simulink model "RBCM_Model"  (R2023b)
settings: Solver=FixedStepAuto  StartTime=0.0  StopTime=10.0  RelTol=1e-3
PreLoadFcn:
  | % NXP_MBDT_S32K3 callback: DO NOT REMOVE
  | mbd_s32k3.common.nxp.model_callbacks.preLoadFcn();
PostLoadFcn:
  | % NXP_MBDT_S32K3 callback: DO NOT REMOVE
  | mbd_s32k3.common.nxp.model_callbacks.postLoadFcn();
InitFcn:
  | % NXP_MBDT_S32K3 callback: DO NOT REMOVE
  | mbd_s32k3.common.nxp.model_callbacks.initFcn();
undefined symbols (not defined in the file or in its folder): AccuFanPwr_hHsd3ch2, BspdPwr_lHsd1ch2, BuzzerPwr_lHsd3ch3, DevicePwr_12v_lHsd1ch1, DevicePwr_hHsd1ch2, DrsPwr_8v_lHsd3ch1, hHsd_Diagnose_AdcBuffer, ILPwr_hHsd1ch1, lHsd_Diagnose_AdcBuffer, LoggerPwr_lHsd1ch3, PumpFan1_hHsd4ch1, PumpFan2_hHsd4ch2, PumpPwr_hHsd3ch1, RGBLED0state, TaillightPwr_lHsd3ch4, TempSensorPwr_lHsd1ch4
libraries: mbd_s32k3_io_library x127, simulink x48, canmsglib x8, mbd_s32k3_communication_library x7, mbd_s32k3_isr_library x6, mbd_s32k3_cdd_library x3, mbd_s32k3_utility_library x1
(part 7 of 9)

== system RBCM_Model/HSD诊断分析子系统/Subsystem2 ==
  u1 : Inport
  Constant : Constant  Value=0xff  OutDataTypeStr=uint8
  Constant2 : Constant  Value=0  OutDataTypeStr=uint8
  Constant3 : Constant  OutDataTypeStr=uint8
  Constant4 : Constant  Value=2  OutDataTypeStr=uint8
  Gain : Gain  Gain=100
  Multiport Switch : MultiPortSwitch  DataPortOrder=Specify indices  DataPortIndices={0,5,90}  DataPortForDefault=Additional data port  DiagnosticForDefault=Warning  SaturateOnIntegerOverflow=off  InputSameDT=off
  u : Outport
  wires:
  Constant4/1 -> Multiport Switch/4
  Constant3/1 -> Multiport Switch/3
  Constant2/1 -> Multiport Switch/2
  Constant/1 -> Multiport Switch/5
  Multiport Switch/1 -> u/1
  Gain/1 -> Multiport Switch/1
  u1/1 -> Gain/1

== system RBCM_Model/HSD诊断分析子系统/Subsystem3 ==
  u1 : Inport
  Constant : Constant  Value=0xff  OutDataTypeStr=uint8
  Constant2 : Constant  Value=0  OutDataTypeStr=uint8
  Constant3 : Constant  OutDataTypeStr=uint8
  Constant4 : Constant  Value=2  OutDataTypeStr=uint8
  Gain : Gain  Gain=100
  Multiport Switch : MultiPortSwitch  DataPortOrder=Specify indices  DataPortIndices={0,5,90}  DataPortForDefault=Additional data port  DiagnosticForDefault=Warning  SaturateOnIntegerOverflow=off  InputSameDT=off
  u : Outport
  wires:
  Constant4/1 -> Multiport Switch/4
  Constant3/1 -> Multiport Switch/3
  Constant2/1 -> Multiport Switch/2
  Constant/1 -> Multiport Switch/5
  Multiport Switch/1 -> u/1
  Gain/1 -> Multiport Switch/1
  u1/1 -> Gain/1

== system RBCM_Model/HSD诊断分析子系统/Subsystem4 ==
  u1 : Inport
  Constant : Constant  Value=0xff  OutDataTypeStr=uint8
  Constant2 : Constant  Value=0  OutDataTypeStr=uint8
  Constant3 : Constant  OutDataTypeStr=uint8
  Constant4 : Constant  Value=2  OutDataTypeStr=uint8
  Gain : Gain  Gain=100
  Multiport Switch : MultiPortSwitch  DataPortOrder=Specify indices  DataPortIndices={0,5,90}  DataPortForDefault=Additional data port  DiagnosticForDefault=Warning  SaturateOnIntegerOverflow=off  InputSameDT=off
  u : Outport
  wires:
  u1/1 -> Gain/1
  Gain/1 -> Multiport Switch/1
  Multiport Switch/1 -> u/1
  Constant/1 -> Multiport Switch/5
  Constant2/1 -> Multiport Switch/2
  Constant3/1 -> Multiport Switch/3
  Constant4/1 -> Multiport Switch/4

== system RBCM_Model/HSD诊断分析子系统/Subsystem5 ==
  u1 : Inport
  Constant : Constant  Value=0xff  OutDataTypeStr=uint8
  Constant2 : Constant  Value=0  OutDataTypeStr=uint8
  Constant3 : Constant  OutDataTypeStr=uint8
  Constant4 : Constant  Value=2  OutDataTypeStr=uint8
  Gain : Gain  Gain=100
  Multiport Switch : MultiPortSwitch  DataPortOrder=Specify indices  DataPortIndices={0,5,90}  DataPortForDefault=Additional data port  DiagnosticForDefault=Warning  SaturateOnIntegerOverflow=off  InputSameDT=off
  u : Outport
  wires:
  Constant4/1 -> Multiport Switch/4
  Constant3/1 -> Multiport Switch/3
  Constant2/1 -> Multiport Switch/2
  Constant/1 -> Multiport Switch/5
  Multiport Switch/1 -> u/1
  Gain/1 -> Multiport Switch/1
  u1/1 -> Gain/1

== system RBCM_Model/HSD诊断分析子系统/Subsystem6 ==
  u1 : Inport
  Constant : Constant  Value=0xff  OutDataTypeStr=uint8
  Constant2 : Constant  Value=0  OutDataTypeStr=uint8
  Constant3 : Constant  OutDataTypeStr=uint8
  Constant4 : Constant  Value=2  OutDataTypeStr=uint8
  Gain : Gain  Gain=100
  Multiport Switch : MultiPortSwitch  DataPortOrder=Specify indices  DataPortIndices={0,5,290}  DataPortForDefault=Additional data port  DiagnosticForDefault=Warning  SaturateOnIntegerOverflow=off  InputSameDT=off
  u : Outport
  wires:
  u1/1 -> Gain/1
  Gain/1 -> Multiport Switch/1
  Multiport Switch/1 -> u/1
  Constant/1 -> Multiport Switch/5
  Constant2/1 -> Multiport Switch/2
  Constant3/1 -> Multiport Switch/3
  Constant4/1 -> Multiport Switch/4

== system RBCM_Model/HSD诊断分析子系统/Subsystem7 ==
  u1 : Inport
  Constant : Constant  Value=0xff  OutDataTypeStr=uint8
  Constant2 : Constant  Value=0  OutDataTypeStr=uint8
  Constant3 : Constant  OutDataTypeStr=uint8
  Constant4 : Constant  Value=2  OutDataTypeStr=uint8
  Gain : Gain  Gain=100
  Multiport Switch : MultiPortSwitch  DataPortOrder=Specify indices  DataPortIndices={0,5,290}  DataPortForDefault=Additional data port  DiagnosticForDefault=Warning  SaturateOnIntegerOverflow=off  InputSameDT=off
  u : Outport
  wires:
  u1/1 -> Gain/1
  Gain/1 -> Multiport Switch/1
  Multiport Switch/1 -> u/1
  Constant/1 -> Multiport Switch/5
  Constant2/1 -> Multiport Switch/2
  Constant3/1 -> Multiport Switch/3
  Constant4/1 -> Multiport Switch/4

== system RBCM_Model/HSD诊断分析子系统/Subsystem8 ==
  u1 : Inport
  Constant : Constant  Value=0xff  OutDataTypeStr=uint8
  Constant2 : Constant  Value=0  OutDataTypeStr=uint8
  Constant3 : Constant  OutDataTypeStr=uint8
  Constant4 : Constant  Value=2  OutDataTypeStr=uint8
  Gain : Gain  Gain=100
  Multiport Switch : MultiPortSwitch  DataPortOrder=Specify indices  DataPortIndices={0,5,290}  DataPortForDefault=Additional data port  DiagnosticForDefault=Warning  SaturateOnIntegerOverflow=off  InputSameDT=off
  u : Outport
  wires:
  Constant4/1 -> Multiport Switch/4
  Constant3/1 -> Multiport Switch/3
  Constant2/1 -> Multiport Switch/2
  Constant/1 -> Multiport Switch/5
  Multiport Switch/1 -> u/1
  Gain/1 -> Multiport Switch/1
  u1/1 -> Gain/1

== system RBCM_Model/HSD诊断分析子系统/Subsystem9 ==
  u1 : Inport
  Constant : Constant  Value=0xff  OutDataTypeStr=uint8
  Constant2 : Constant  Value=0  OutDataTypeStr=uint8
  Constant3 : Constant  OutDataTypeStr=uint8
  Constant4 : Constant  Value=2  OutDataTypeStr=uint8
  Gain : Gain  Gain=100
  Multiport Switch : MultiPortSwitch  DataPortOrder=Specify indices  DataPortIndices={0,5,290}  DataPortForDefault=Additional data port  DiagnosticForDefault=Warning  SaturateOnIntegerOverflow=off  InputSameDT=off
  u : Outport
  wires:
  u1/1 -> Gain/1
  Gain/1 -> Multiport Switch/1
  Multiport Switch/1 -> u/1
  Constant/1 -> Multiport Switch/5
  Constant2/1 -> Multiport Switch/2
  Constant3/1 -> Multiport Switch/3
  Constant4/1 -> Multiport Switch/4

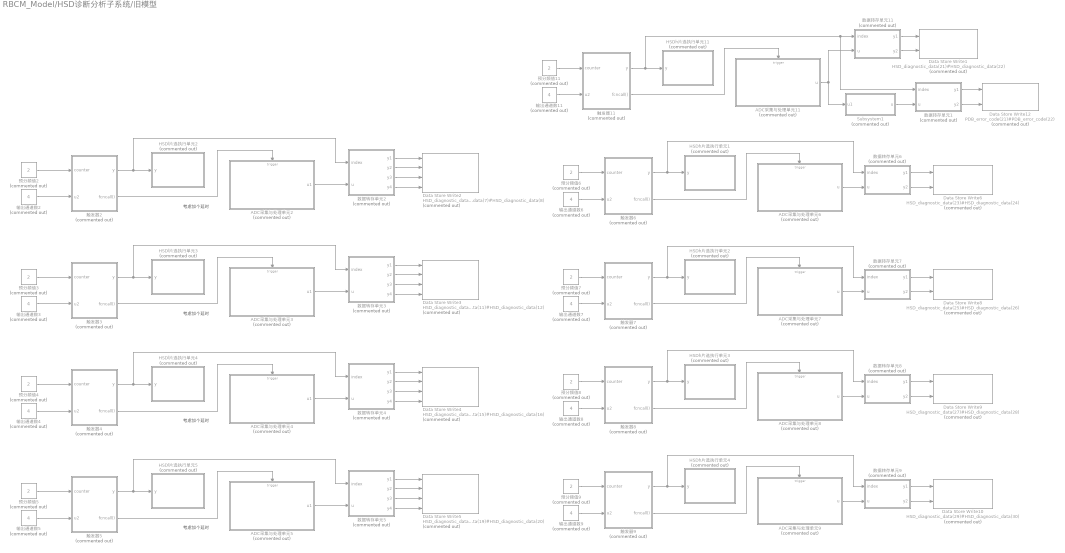
== system RBCM_Model/HSD诊断分析子系统/旧模型 ==
  note: 考虑加个延时
  note: 考虑加个延时
  note: 考虑加个延时
  note: 考虑加个延时
  ADC采集与处理单元11 : Subsystem  Commented=on
  ADC采集与处理单元2 : Subsystem  Commented=on
  ADC采集与处理单元3 : Subsystem  Commented=on
  ADC采集与处理单元4 : Subsystem  Commented=on
  ADC采集与处理单元5 : Subsystem  Commented=on
  ADC采集与处理单元6 : Subsystem  Commented=on
  ADC采集与处理单元7 : Subsystem  Commented=on
  ADC采集与处理单元8 : Subsystem  Commented=on
  ADC采集与处理单元9 : Subsystem  Commented=on
  Data Store Write1 : DataStoreWrite  Commented=on  DataStoreName=HSD_diagnostic_data  DataStoreElements=HSD_diagnostic_data(21)#HSD_diagnostic_data(22)  IndexOptions=Index vector (dialog)  Indices=1  OutputSizes=1
  Data Store Write10 : DataStoreWrite  Commented=on  DataStoreName=HSD_diagnostic_data  DataStoreElements=HSD_diagnostic_data(29)#HSD_diagnostic_data(30)  IndexOptions=Index vector (dialog)  Indices=1  OutputSizes=1
  Data Store Write12 : DataStoreWrite  Commented=on  DataStoreName=PDB_error_code  DataStoreElements=PDB_error_code(21)#PDB_error_code(22)  IndexOptions=Index vector (dialog)  Indices=1  OutputSizes=1
  Data Store Write2 : DataStoreWrite  Commented=on  DataStoreName=HSD_diagnostic_data  DataStoreElements=HSD_diagnostic_data(5)#HSD_diagnostic_data(6)#HSD_diagnostic_data(7)#HSD_diagnostic_data(8)  IndexOptions=Index vector (dialog)  Indices=1  OutputSizes=1
  Data Store Write3 : DataStoreWrite  Commented=on  DataStoreName=HSD_diagnostic_data  DataStoreElements=HSD_diagnostic_data(9)#HSD_diagnostic_data(10)#HSD_diagnostic_data(11)#HSD_diagnostic_data(12)  IndexOptions=Index vector (dialog)  Indices=1  OutputSizes=1
  Data Store Write4 : DataStoreWrite  Commented=on  DataStoreName=HSD_diagnostic_data  DataStoreElements=HSD_diagnostic_data(13)#HSD_diagnostic_data(14)#HSD_diagnostic_data(15)#HSD_diagnostic_data(16)  IndexOptions=Index vector (dialog)  Indices=1  OutputSizes=1
  Data Store Write5 : DataStoreWrite  Commented=on  DataStoreName=HSD_diagnostic_data  DataStoreElements=HSD_diagnostic_data(17)#HSD_diagnostic_data(18)#HSD_diagnostic_data(19)#HSD_diagnostic_data(20)  IndexOptions=Index vector (dialog)  Indices=1  OutputSizes=1
  Data Store Write6 : DataStoreWrite  Commented=on  DataStoreName=HSD_diagnostic_data  DataStoreElements=HSD_diagnostic_data(23)#HSD_diagnostic_data(24)  IndexOptions=Index vector (dialog)  Indices=1  OutputSizes=1
  Data Store Write8 : DataStoreWrite  Commented=on  DataStoreName=HSD_diagnostic_data  DataStoreElements=HSD_diagnostic_data(25)#HSD_diagnostic_data(26)  IndexOptions=Index vector (dialog)  Indices=1  OutputSizes=1
  Data Store Write9 : DataStoreWrite  Commented=on  DataStoreName=HSD_diagnostic_data  DataStoreElements=HSD_diagnostic_data(27)#HSD_diagnostic_data(28)  IndexOptions=Index vector (dialog)  Indices=1  OutputSizes=1
  HSDh片选执行单元1 : Subsystem  Commented=on
  HSDh片选执行单元11 : Subsystem  Commented=on
  HSDh片选执行单元2 : Subsystem  Commented=on
  HSDh片选执行单元3 : Subsystem  Commented=on
  HSDh片选执行单元4 : Subsystem  Commented=on
  HSDl片选执行单元2 : Subsystem  Commented=on
  HSDl片选执行单元3 : Subsystem  Commented=on
  HSDl片选执行单元4 : Subsystem  Commented=on
  HSDl片选执行单元5 : Subsystem  Commented=on
  Subsystem1 : Subsystem  Commented=on
  数据转存单元1 : MATLAB Function  Commented=on  TreatAsAtomicUnit=on
  数据转存单元11 : MATLAB Function  Commented=on  TreatAsAtomicUnit=on
  数据转存单元2 : MATLAB Function  Commented=on  TreatAsAtomicUnit=on
  数据转存单元3 : MATLAB Function  Commented=on  TreatAsAtomicUnit=on
  数据转存单元4 : MATLAB Function  Commented=on  TreatAsAtomicUnit=on
  数据转存单元5 : MATLAB Function  Commented=on  TreatAsAtomicUnit=on
  数据转存单元6 : MATLAB Function  Commented=on  TreatAsAtomicUnit=on
  数据转存单元7 : MATLAB Function  Commented=on  TreatAsAtomicUnit=on
  数据转存单元8 : MATLAB Function  Commented=on  TreatAsAtomicUnit=on
  数据转存单元9 : MATLAB Function  Commented=on  TreatAsAtomicUnit=on
  触发器11 : MATLAB Function  Commented=on  TreatAsAtomicUnit=on
  触发器2 : MATLAB Function  Commented=on  TreatAsAtomicUnit=on
  触发器3 : MATLAB Function  Commented=on  TreatAsAtomicUnit=on
  触发器4 : MATLAB Function  Commented=on  TreatAsAtomicUnit=on
  触发器5 : MATLAB Function  Commented=on  TreatAsAtomicUnit=on
  触发器6 : MATLAB Function  Commented=on  TreatAsAtomicUnit=on
  触发器7 : MATLAB Function  Commented=on  TreatAsAtomicUnit=on
  触发器8 : MATLAB Function  Commented=on  TreatAsAtomicUnit=on
  触发器9 : MATLAB Function  Commented=on  TreatAsAtomicUnit=on
  输出通道数{2..9,11} (9 alike) : Constant  Commented=on  Value=4  OutDataTypeStr=uint8
  预分频值{2..9,11} (9 alike) : Constant  Commented=on  Value=2  OutDataTypeStr=uint8
  wires:
  预分频值7/1 -> 触发器7/1(counter)
  ADC采集与处理单元3/1(u1) -> 数据转存单元3/2(u)
  输出通道数4/1 -> 触发器4/2(u2)
  触发器6/1(y) -> 数据转存单元6/1(index), HSDh片选执行单元1/1(y)
  预分频值8/1 -> 触发器8/1(counter)
  数据转存单元4/2(y2) -> Data Store Write4/2
  触发器8/1(y) -> 数据转存单元8/1(index), HSDh片选执行单元3/1(y)
  触发器7/2(fcncall()) -> ADC采集与处理单元7/Trigger
  数据转存单元3/4(y4) -> Data Store Write3/4
  数据转存单元3/1(y1) -> Data Store Write3/1
  数据转存单元4/3(y3) -> Data Store Write4/3
  触发器6/2(fcncall()) -> ADC采集与处理单元6/Trigger
  预分频值2/1 -> 触发器2/1(counter)
  预分频值6/1 -> 触发器6/1(counter)
  数据转存单元2/2(y2) -> Data Store Write2/2
  ADC采集与处理单元4/1(u1) -> 数据转存单元4/2(u)
  输出通道数8/1 -> 触发器8/2(u2)
  触发器2/2(fcncall()) -> ADC采集与处理单元2/Trigger
  输出通道数3/1 -> 触发器3/2(u2)
  数据转存单元2/1(y1) -> Data Store Write2/1
  触发器7/1(y) -> HSDh片选执行单元2/1(y), 数据转存单元7/1(index)
  触发器3/1(y) -> HSDl片选执行单元3/1(y), 数据转存单元3/1(index)
  输出通道数7/1 -> 触发器7/2(u2)
  触发器5/1(y) -> HSDl片选执行单元5/1(y), 数据转存单元5/1(index)
  触发器8/2(fcncall()) -> ADC采集与处理单元8/Trigger
  预分频值5/1 -> 触发器5/1(counter)
  ADC采集与处理单元5/1(u1) -> 数据转存单元5/2(u)
  数据转存单元6/1(y1) -> Data Store Write6/1
  预分频值4/1 -> 触发器4/1(counter)
  预分频值3/1 -> 触发器3/1(counter)
  数据转存单元3/2(y2) -> Data Store Write3/2
  数据转存单元7/2(y2) -> Data Store Write8/2
  输出通道数6/1 -> 触发器6/2(u2)
  触发器4/1(y) -> 数据转存单元4/1(index), HSDl片选执行单元4/1(y)
  输出通道数5/1 -> 触发器5/2(u2)
  数据转存单元9/2(y2) -> Data Store Write10/2
  ADC采集与处理单元8/1(u) -> 数据转存单元8/2(u)
  数据转存单元2/4(y4) -> Data Store Write2/4
  数据转存单元5/1(y1) -> Data Store Write5/1
  触发器2/1(y) -> 数据转存单元2/1(index), HSDl片选执行单元2/1(y)
  数据转存单元3/3(y3) -> Data Store Write3/3
  输出通道数2/1 -> 触发器2/2(u2)
  数据转存单元5/4(y4) -> Data Store Write5/4
  预分频值9/1 -> 触发器9/1(counter)
  数据转存单元2/3(y3) -> Data Store Write2/3
  ADC采集与处理单元2/1(u1) -> 数据转存单元2/2(u)
  ADC采集与处理单元9/1(u) -> 数据转存单元9/2(u)
  数据转存单元6/2(y2) -> Data Store Write6/2
  触发器4/2(fcncall()) -> ADC采集与处理单元4/Trigger
  ADC采集与处理单元6/1(u) -> 数据转存单元6/2(u)
  数据转存单元4/4(y4) -> Data Store Write4/4
  数据转存单元5/2(y2) -> Data Store Write5/2
  输出通道数9/1 -> 触发器9/2(u2)
  数据转存单元8/2(y2) -> Data Store Write9/2
  触发器9/1(y) -> HSDh片选执行单元4/1(y), 数据转存单元9/1(index)
  触发器5/2(fcncall()) -> ADC采集与处理单元5/Trigger
  触发器3/2(fcncall()) -> ADC采集与处理单元3/Trigger
  数据转存单元4/1(y1) -> Data Store Write4/1
  数据转存单元9/1(y1) -> Data Store Write10/1
  ADC采集与处理单元7/1(u) -> 数据转存单元7/2(u)
  数据转存单元7/1(y1) -> Data Store Write8/1
  数据转存单元8/1(y1) -> Data Store Write9/1
  触发器9/2(fcncall()) -> ADC采集与处理单元9/Trigger
  数据转存单元5/3(y3) -> Data Store Write5/3
  触发器11/2(fcncall()) -> ADC采集与处理单元11/Trigger
  数据转存单元1/2(y2) -> Data Store Write12/2
  Subsystem1/1(u) -> 数据转存单元1/2(u)
  数据转存单元11/2(y2) -> Data Store Write1/2
  数据转存单元11/1(y1) -> Data Store Write1/1
  输出通道数11/1 -> 触发器11/2(u2)
  预分频值11/1 -> 触发器11/1(counter)
  数据转存单元1/1(y1) -> Data Store Write12/1
  触发器11/1(y) -> HSDh片选执行单元11/1(y), 数据转存单元1/1(index), 数据转存单元11/1(index)
  ADC采集与处理单元11/1(u) -> Subsystem1/1(u1), 数据转存单元11/2(u)

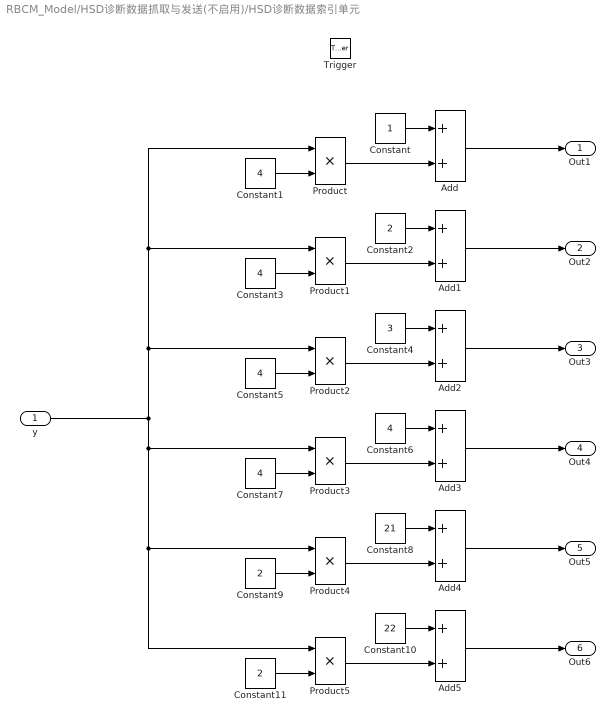
== system RBCM_Model/HSD诊断数据抓取与发送(不启用)/HSD诊断数据索引单元 ==
  y : Inport  OutDataTypeStr=uint8
  Trigger : TriggerPort  TriggerType=function-call  VariantControl=(inherit)  PortDimensions=1
  Add{,1..5} (6 alike) : Sum  OutDataTypeStr=uint8
  Constant : Constant  OutDataTypeStr=uint8
  Constant{1,3,5..7} (5 alike) : Constant  Value=4  OutDataTypeStr=uint8
  Constant10 : Constant  Value=22  OutDataTypeStr=uint8
  Constant11 : Constant  Value=2  OutDataTypeStr=uint8
  Constant2 : Constant  Value=2  OutDataTypeStr=uint8
  Constant4 : Constant  Value=3  OutDataTypeStr=uint8
  Constant8 : Constant  Value=21  OutDataTypeStr=uint8
  Constant9 : Constant  Value=2  OutDataTypeStr=uint8
  Product{,1..5} (6 alike) : Product  OutDataTypeStr=uint8
  Out1 : Outport  OutDataTypeStr=uint8
  Out2 : Outport  Port=2  OutDataTypeStr=uint8
  Out3 : Outport  Port=3  OutDataTypeStr=uint8
  Out4 : Outport  Port=4  OutDataTypeStr=uint8
  Out5 : Outport  Port=5  OutDataTypeStr=uint8
  Out6 : Outport  Port=6  OutDataTypeStr=uint8
  wires:
  Product/1 -> Add/2
  Constant1/1 -> Product/2
  Add/1 -> Out1/1
  Constant/1 -> Add/1
  Constant2/1 -> Add1/1
  Add1/1 -> Out2/1
  Constant3/1 -> Product1/2
  Product1/1 -> Add1/2
  Product3/1 -> Add3/2
  Constant7/1 -> Product3/2
  Add3/1 -> Out4/1
  Constant6/1 -> Add3/1
  Constant4/1 -> Add2/1
  Add2/1 -> Out3/1
  Constant5/1 -> Product2/2
  Product2/1 -> Add2/2
  Product4/1 -> Add4/2
  Constant9/1 -> Product4/2
  Add4/1 -> Out5/1
  Constant8/1 -> Add4/1
  Constant10/1 -> Add5/1
  Add5/1 -> Out6/1
  Constant11/1 -> Product5/2
  Product5/1 -> Add5/2
  y/1 -> Product5/1, Product4/1, Product3/1, Product2/1, Product1/1, Product/1

== system RBCM_Model/HSD驱动子系统/HSDh输出控制单元1 ==
  In1 : Inport
  In2 : Inport  Port=2
  Dio : mbd_s32k3_io_library/Dio  Commented=on  api_func=Dio_WriteChannel  channel=RGBLED0_BLUE  channel_group=No channel groups configured  port=PTB_H  gpioSim=on  text=<binary blob, 15246 chars, not shown>
      settings: SourceProductName=NXP Model-Based Design Toolbox for S32K3 MCUs
  Dio1 : mbd_s32k3_io_library/Dio  api_func=Dio_WriteChannel  channel=RGBLED0_BLUE  channel_group=No channel groups configured  port=PTB_H  gpioSim=on  text=<binary blob, 15399 chars, not shown>
      settings: SourceProductName=NXP Model-Based Design Toolbox for S32K3 MCUs
  wires:
  In2/1 -> Dio1/1
  In1/1 -> Dio/1

== system RBCM_Model/HSD驱动子系统/HSDh输出控制单元2 ==
  note: PUMP_PWM_CTRL
  In1 : Inport  OutDataTypeStr=uint8
  In2 : Inport  Port=2  OutDataTypeStr=uint8
  Dio : mbd_s32k3_io_library/Dio  api_func=Dio_WriteChannel  channel=RGBLED0_BLUE  channel_group=No channel groups configured  port=PTB_H  gpioSim=on  text=<binary blob, 15399 chars, not shown>
      settings: SourceProductName=NXP Model-Based Design Toolbox for S32K3 MCUs
  Dio1 : mbd_s32k3_io_library/Dio  api_func=Dio_WriteChannel  channel=RGBLED0_BLUE  channel_group=No channel groups configured  port=PTB_H  gpioSim=on  text=<binary blob, 15399 chars, not shown>
      settings: SourceProductName=NXP Model-Based Design Toolbox for S32K3 MCUs
  wires:
  In2/1 -> Dio1/1
  In1/1 -> Dio/1

== system RBCM_Model/HSD驱动子系统/HSDh输出控制单元3 ==
  note: FAN1_PWM_CTRL
  In1 : Inport
  In2 : Inport  Port=2
  Dio : mbd_s32k3_io_library/Dio  api_func=Dio_WriteChannel  channel=RGBLED0_BLUE  channel_group=No channel groups configured  port=PTB_H  gpioSim=on  text=<binary blob, 15399 chars, not shown>
      settings: SourceProductName=NXP Model-Based Design Toolbox for S32K3 MCUs
  Dio1 : mbd_s32k3_io_library/Dio  api_func=Dio_WriteChannel  channel=RGBLED0_BLUE  channel_group=No channel groups configured  port=PTB_H  gpioSim=on  text=<binary blob, 15399 chars, not shown>
      settings: SourceProductName=NXP Model-Based Design Toolbox for S32K3 MCUs
  wires:
  In2/1 -> Dio1/1
  In1/1 -> Dio/1

== system RBCM_Model/HSD驱动子系统/HSDh输出控制单元4 ==
  note: FAN1_PWM_CTRL
  In1 : Inport
  In2 : Inport  Port=2
  Dio : mbd_s32k3_io_library/Dio  api_func=Dio_WriteChannel  channel=RGBLED0_BLUE  channel_group=No channel groups configured  port=PTB_H  gpioSim=on  text=<binary blob, 15399 chars, not shown>
      settings: SourceProductName=NXP Model-Based Design Toolbox for S32K3 MCUs
  Dio1 : mbd_s32k3_io_library/Dio  api_func=Dio_WriteChannel  channel=RGBLED0_BLUE  channel_group=No channel groups configured  port=PTB_H  gpioSim=on  text=<binary blob, 15399 chars, not shown>
      settings: SourceProductName=NXP Model-Based Design Toolbox for S32K3 MCUs
  wires:
  In2/1 -> Dio1/1
  In1/1 -> Dio/1

== system RBCM_Model/HSD驱动子系统/HSDh输出控制单元5 ==
  In1 : Inport
  In2 : Inport  Port=2
  Dio : mbd_s32k3_io_library/Dio  api_func=Dio_WriteChannel  channel=RGBLED0_BLUE  channel_group=No channel groups configured  port=PTB_H  gpioSim=on  text=<binary blob, 15399 chars, not shown>
      settings: SourceProductName=NXP Model-Based Design Toolbox for S32K3 MCUs
  Dio1 : mbd_s32k3_io_library/Dio  api_func=Dio_WriteChannel  channel=RGBLED0_BLUE  channel_group=No channel groups configured  port=PTB_H  gpioSim=on  text=<binary blob, 15399 chars, not shown>
      settings: SourceProductName=NXP Model-Based Design Toolbox for S32K3 MCUs
  wires:
  In2/1 -> Dio1/1
  In1/1 -> Dio/1

== system RBCM_Model/HSD驱动子系统/HSDh输出控制单元6 ==
  In1 : Inport
  In2 : Inport  Port=2
  Dio : mbd_s32k3_io_library/Dio  api_func=Dio_WriteChannel  channel=RGBLED0_BLUE  channel_group=No channel groups configured  port=PTB_H  gpioSim=on  text=<binary blob, 15399 chars, not shown>
      settings: SourceProductName=NXP Model-Based Design Toolbox for S32K3 MCUs
  Dio1 : mbd_s32k3_io_library/Dio  api_func=Dio_WriteChannel  channel=RGBLED0_BLUE  channel_group=No channel groups configured  port=PTB_H  gpioSim=on  text=<binary blob, 15399 chars, not shown>
      settings: SourceProductName=NXP Model-Based Design Toolbox for S32K3 MCUs
  wires:
  In1/1 -> Dio/1
  In2/1 -> Dio1/1

== system RBCM_Model/HSD驱动子系统/HSDl输出控制单元1 ==
  In1 : Inport
  In2 : Inport  Port=2
  In3 : Inport  Port=3
  In6 : Inport  Port=4
  Dio{,1..3} (4 alike) : mbd_s32k3_io_library/Dio  api_func=Dio_WriteChannel  channel=RGBLED0_BLUE  channel_group=No channel groups configured  port=PTB_H  gpioSim=on  text=<binary blob, 15399 chars, not shown>
      settings: SourceProductName=NXP Model-Based Design Toolbox for S32K3 MCUs
  wires:
  In6/1 -> Dio3/1
  In2/1 -> Dio1/1
  In3/1 -> Dio2/1
  In1/1 -> Dio/1

== system RBCM_Model/HSD驱动子系统/HSDl输出控制单元2 ==
  In1 : Inport
  In2 : Inport  Port=2
  In3 : Inport  Port=3
  In6 : Inport  Port=4
  Dio{,1,3..4} (4 alike) : mbd_s32k3_io_library/Dio  api_func=Dio_WriteChannel  channel=RGBLED0_BLUE  channel_group=No channel groups configured  port=PTB_H  gpioSim=on  text=<binary blob, 15399 chars, not shown>
      settings: SourceProductName=NXP Model-Based Design Toolbox for S32K3 MCUs
  wires:
  In1/1 -> Dio/1
  In3/1 -> Dio4/1
  In2/1 -> Dio1/1
  In6/1 -> Dio3/1

== system RBCM_Model/HSD驱动子系统/HSDl输出控制单元3 ==
  In1 : Inport
  In2 : Inport  Port=2
  In3 : Inport  Port=3
  In6 : Inport  Port=4
  Dio{,1..3} (4 alike) : mbd_s32k3_io_library/Dio  api_func=Dio_WriteChannel  channel=RGBLED0_BLUE  channel_group=No channel groups configured  port=PTB_H  gpioSim=on  text=<binary blob, 15399 chars, not shown>
      settings: SourceProductName=NXP Model-Based Design Toolbox for S32K3 MCUs
  wires:
  In6/1 -> Dio3/1
  In2/1 -> Dio1/1
  In3/1 -> Dio2/1
  In1/1 -> Dio/1

== system RBCM_Model/HSD驱动子系统/HSDl输出控制单元4 ==
  In1 : Inport
  In2 : Inport  Port=2
  In3 : Inport  Port=3
  In6 : Inport  Port=4
  Dio{,1..3} (4 alike) : mbd_s32k3_io_library/Dio  api_func=Dio_WriteChannel  channel=RGBLED0_BLUE  channel_group=No channel groups configured  port=PTB_H  gpioSim=on  text=<binary blob, 15399 chars, not shown>
      settings: SourceProductName=NXP Model-Based Design Toolbox for S32K3 MCUs
  wires:
  In1/1 -> Dio/1
  In3/1 -> Dio2/1
  In2/1 -> Dio1/1
  In6/1 -> Dio3/1

== system RBCM_Model/HSD驱动子系统/HSDl输出控制单元5 ==
  In1 : Inport
  In2 : Inport  Port=2
  In3 : Inport  Port=3
  In6 : Inport  Port=4
  Dio{,1..3} (4 alike) : mbd_s32k3_io_library/Dio  api_func=Dio_WriteChannel  channel=RGBLED0_BLUE  channel_group=No channel groups configured  port=PTB_H  gpioSim=on  text=<binary blob, 15399 chars, not shown>
      settings: SourceProductName=NXP Model-Based Design Toolbox for S32K3 MCUs
  wires:
  In6/1 -> Dio3/1
  In2/1 -> Dio1/1
  In3/1 -> Dio2/1
  In1/1 -> Dio/1

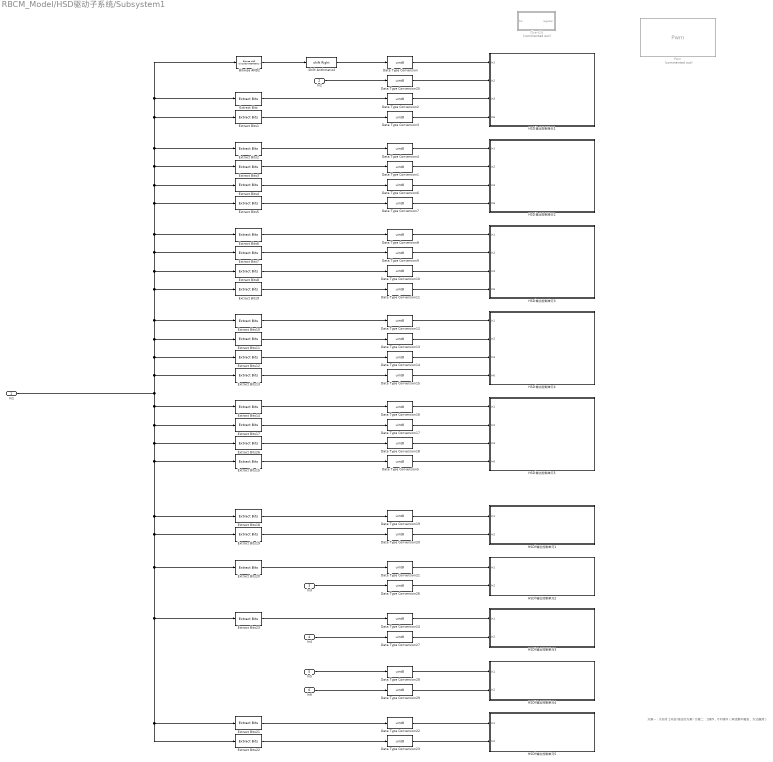
== system RBCM_Model/HSD驱动子系统/Subsystem1 ==
  note: 方案一：0关闭 1开启(现在的方案)
      | 方案二：1操作，0不操作（异或集中触发，方式最简）
  In1 : Inport  OutDataTypeStr=uint32
  In2 : Inport  Port=2  OutDataTypeStr=uint8
  In3 : Inport  Port=3  OutDataTypeStr=uint8
  In4 : Inport  Port=4  OutDataTypeStr=uint8
  In5 : Inport  Port=5  OutDataTypeStr=uint8
  In6 : Inport  Port=6  OutDataTypeStr=uint8
  Bitwise AND2 : simulink/Logic and Bit Operations/Bitwise Operator  logicop=AND  UseBitMask=on  BitMask=bin2dec('00000001')  BitMaskRealWorld=Stored Integer
      settings: LibrarySourceBlock=|
      | simulink/Quick Insert/Logic and Bit
      | Operations/Bitwise AND
  Chart19 : Stateflow chart  Commented=on  TreatAsAtomicUnit=on
  Data Type Conversion{,1..29} (30 alike) : DataTypeConversion  OutDataTypeStr=uint8  SaturateOnIntegerOverflow=off  RndMeth=Floor
  Extract Bits : simulink/Logic and Bit Operations/Extract Bits  bitsToExtract=Range of bits  numBits=8  bitIdxRange=[2 2]  outScalingMode=Preserve fixed-point scaling
  Extract Bits1 : simulink/Logic and Bit Operations/Extract Bits  bitsToExtract=Range of bits  numBits=8  bitIdxRange=[3 3]  outScalingMode=Preserve fixed-point scaling
  Extract Bits10 : simulink/Logic and Bit Operations/Extract Bits  bitsToExtract=Range of bits  numBits=8  bitIdxRange=[24 25]  outScalingMode=Preserve fixed-point scaling
  Extract Bits11 : simulink/Logic and Bit Operations/Extract Bits  bitsToExtract=Range of bits  numBits=8  bitIdxRange=[26 27]  outScalingMode=Preserve fixed-point scaling
  Extract Bits12 : simulink/Logic and Bit Operations/Extract Bits  bitsToExtract=Range of bits  numBits=8  bitIdxRange=[28 29]  outScalingMode=Preserve fixed-point scaling
  Extract Bits13 : simulink/Logic and Bit Operations/Extract Bits  bitsToExtract=Range of bits  numBits=8  bitIdxRange=[30 31]  outScalingMode=Preserve fixed-point scaling
  Extract Bits14 : simulink/Logic and Bit Operations/Extract Bits  bitsToExtract=Range of bits  numBits=8  bitIdxRange=[32 33]  outScalingMode=Preserve fixed-point scaling
  Extract Bits{15,18..23,26} (8 alike) : simulink/Logic and Bit Operations/Extract Bits  bitsToExtract=Range of bits  numBits=8  bitIdxRange=[36 37]  outScalingMode=Preserve fixed-point scaling
  Extract Bits17 : simulink/Logic and Bit Operations/Extract Bits  bitsToExtract=Range of bits  numBits=8  bitIdxRange=[34 35]  outScalingMode=Preserve fixed-point scaling
  Extract Bits2 : simulink/Logic and Bit Operations/Extract Bits  bitsToExtract=Range of bits  numBits=8  bitIdxRange=[4 4]  outScalingMode=Preserve fixed-point scaling
  Extract Bits3 : simulink/Logic and Bit Operations/Extract Bits  bitsToExtract=Range of bits  numBits=8  bitIdxRange=[5 5]  outScalingMode=Preserve fixed-point scaling
  Extract Bits4 : simulink/Logic and Bit Operations/Extract Bits  bitsToExtract=Range of bits  numBits=8  bitIdxRange=[6 6]  outScalingMode=Preserve fixed-point scaling
  Extract Bits5 : simulink/Logic and Bit Operations/Extract Bits  bitsToExtract=Range of bits  numBits=8  bitIdxRange=[7 7]  outScalingMode=Preserve fixed-point scaling
  Extract Bits6 : simulink/Logic and Bit Operations/Extract Bits  bitsToExtract=Range of bits  numBits=8  bitIdxRange=[16 17]  outScalingMode=Preserve fixed-point scaling
  Extract Bits7 : simulink/Logic and Bit Operations/Extract Bits  bitsToExtract=Range of bits  numBits=8  bitIdxRange=[18 19]  outScalingMode=Preserve fixed-point scaling
  Extract Bits8 : simulink/Logic and Bit Operations/Extract Bits  bitsToExtract=Range of bits  numBits=8  bitIdxRange=[20 21]  outScalingMode=Preserve fixed-point scaling
  Extract Bits9 : simulink/Logic and Bit Operations/Extract Bits  bitsToExtract=Range of bits  numBits=8  bitIdxRange=[22 23]  outScalingMode=Preserve fixed-point scaling
  HSDh输出控制单元1 : Subsystem
  HSDh输出控制单元2 : Subsystem
  HSDh输出控制单元3 : Subsystem
  HSDh输出控制单元4 : Subsystem
  HSDh输出控制单元5 : Subsystem
  HSDl输出控制单元1 : Subsystem
  HSDl输出控制单元2 : Subsystem
  HSDl输出控制单元3 : Subsystem
  HSDl输出控制单元4 : Subsystem
  HSDl输出控制单元5 : Subsystem
  Pwm : mbd_s32k3_io_library/Pwm  Commented=on  api_func=Pwm_SetDutyCycle  channel=PwmChannel_0  notification=PWM_RISING_EDGE  moduleId=PWM_EMIOS_INSTANCE_0  prescalerType=PWM_PRIMARY_PRESCALER  text=|
      | CommonPublishedInformation - CommonPublishedInformation Pwm 
      | CommonPublishedInformation/ArReleaseMajorVersion - 4 
      | CommonPublishedInformation/ArReleaseMinorVersion - 4 
      | CommonPublishedInformation/ArReleaseRevisionVersion - 0 
      | CommonPublishedInformation/ModuleId - 121 
      | CommonPublishedInformation/SwMajorVersion - 2 
      | CommonPublishedInformation/SwMinorVersion - 0 
      | CommonPublishedInformation/SwPatchVersion - 0 
      | CommonPublishedInformation/VendorId - 43 
      | IMPLEMENTATION-CONFIG-VARIANT - VARIANT-POST-BUILD 
      | POST_BUILD_VARIANT_USED - true 
      | PwmChannel - PwmChannel_0 PwmChannel_1 PwmChannel_2 PwmChannel_3 PwmChannel_4 PwmChannel_5 PwmChannel_6 PwmChannel_7 PwmChannel_8 
      | PwmChannel_0/Index - 0 
      | PwmChannel_0/PwmChannelId - 0 
      | PwmChannel_0/PwmDutycycleDefault - 2048 
      | PwmChannel_0/PwmHwChannel - /Pwm/Pwm/PwmChannelConfigSet/PwmEmios_0/PwmEmiosChannels_9 
      | PwmChannel_0/PwmIdleState - PWM_LOW 
      | PwmChannel_0/PwmMcuClockReferencePoint - /Mcu/Mcu/McuModuleConfiguration/McuClockSettingConfig_0/CORE_CLK 
      | PwmChannel_0/PwmNotification - PwmChannel_0_Callback 
      | PwmChannel_0/PwmPeriodDefault - 16000.0 
      | PwmChannel_0/PwmPeriodInTicks - true 
      | PwmChannel_0/PwmPolarity - PWM_HIGH 
      | PwmChannel_1/Index - 1 
      | PwmChannel_1/PwmChannelId - 1 
      | PwmChannel_1/PwmDutycycleDefault - 2048 
      | PwmChannel_1/PwmHwChannel - /Pwm/Pwm/PwmChannelConfigSet/PwmEmios_0/PwmEmiosChannels_17 
      | PwmChannel_1/PwmIdleState - PWM_LOW 
      | PwmChannel_1/PwmMcuClockReferencePoint - /Mcu/Mcu/McuModuleConfiguration/McuClockSettingConfig_0/CORE_CLK 
      | PwmChannel_1/PwmNotification - PwmChannel_1_Callback 
      | PwmChannel_1/PwmPeriodDefault - 16000.0 
      | PwmChannel_1/PwmPeriodInTicks - true 
      | PwmChannel_1/PwmPolarity - PWM_HIGH 
      | PwmChannel_2/Index - 2 
      | PwmChannel_2/PwmChannelId - 2 
      | PwmChannel_2/PwmDutycycleDefault - 0 
      | PwmChannel_2/PwmHwChannel - /Pwm/Pwm/PwmChannelConfigSet/PwmEmios_1/PwmEmiosChannels_19 
      | PwmChannel_2/PwmIdleState - PWM_LOW 
      | PwmChannel_2/PwmMcuClockReferencePoint - /Mcu/Mcu/McuModuleConfiguration/McuClockSettingConfig_0/CORE_CLK 
      | PwmChannel_2/PwmNotification - PwmChannel_2_Callback 
      | PwmChannel_2/PwmPeriodDefault - 16000.0 
      | PwmChannel_2/PwmPeriodInTicks - true 
      | PwmChannel_2/PwmPolarity - PWM_HIGH 
      | PwmChannel_3/Index - 3 
      | PwmChannel_3/PwmChannelId - 3 
      | PwmChannel_3/PwmDutycycleDefault - 0 
      | PwmChannel_3/PwmHwChannel - /Pwm/Pwm/PwmChannelConfigSet/PwmEmios_1/PwmEmiosChannels_20 
      | PwmChannel_3/PwmIdleState - PWM_LOW 
      | PwmChannel_3/PwmMcuClockReferencePoint - /Mcu/Mcu/McuModuleConfiguration/McuClockSettingConfig_0/CORE_CLK 
      | PwmChannel_3/PwmNotification - PwmChannel_3_Callback 
      | PwmChannel_3/PwmPeriodDefault - 16000.0 
      | PwmChannel_3/PwmPeriodInTicks - true 
      | PwmChannel_3/PwmPolarity - PWM_HIGH 
      | PwmChannel_4/Index - 4 
      | PwmChannel_4/PwmChannelId - 4 
      | PwmChannel_4/PwmDutycycleDefault - 0 
      | PwmChannel_4/PwmHwChannel - /Pwm/Pwm/PwmChannelConfigSet/PwmEmios_1/PwmEmiosChannels_0 
      | PwmChannel_4/PwmIdleState - PWM_LOW 
      | PwmChannel_4/PwmMcuClockReferencePoint - /Mcu/Mcu/McuModuleConfiguration/McuClockSettingConfig_0/CORE_CLK 
      | PwmChannel_4/PwmNotification - PwmChannel_4_Callback 
      | PwmChannel_4/PwmPeriodDefault - 16000.0 
      | PwmChannel_4/PwmPeriodInTicks - true 
      | PwmChannel_4/PwmPolarity - PWM_HIGH 
      | PwmChannel_5/Index - 5 
      | PwmChannel_5/PwmChannelId - 5 
      | PwmChannel_5/PwmDutycycleDefault - 0 
      | PwmChannel_5/PwmHwChannel - /Pwm/Pwm/PwmChannelConfigSet/PwmEmios_1/PwmEmiosChannels_1 
      | PwmChannel_5/PwmIdleState - PWM_LOW 
      | PwmChannel_5/PwmMcuClockReferencePoint - /Mcu/Mcu/McuModuleConfiguration/McuClockSettingConfig_0/CORE_CLK 
      | PwmChannel_5/PwmNotification - PwmChannel_5_Callback 
      | PwmChannel_5/PwmPeriodDefault - 16000.0 
      | PwmChannel_5/PwmPeriodInTicks - true 
      | PwmChannel_5/PwmPolarity - PWM_HIGH 
      | PwmChannel_6/Index - 6 
      | PwmChannel_6/PwmChannelId - 6 
      | PwmChannel_6/PwmDutycycleDefault - 0 
      | PwmChannel_6/PwmHwChannel - /Pwm/Pwm/PwmChannelConfigSet/PwmEmios_1/PwmEmiosChannels_21 
      | PwmChannel_6/PwmIdleState - PWM_LOW 
      | PwmChannel_6/PwmMcuClockReferencePoint - /Mcu/Mcu/McuModuleConfiguration/McuClockSettingConfig_0/CORE_CLK 
      | PwmChannel_6/PwmNotification - PwmChannel_6_Callback 
      | PwmChannel_6/PwmPeriodDefault - 16000.0 
      | PwmChannel_6/PwmPeriodInTicks - true 
      | PwmChannel_6/PwmPolarity - PWM_HIGH 
      | PwmChannel_7/Index - 7 
      | PwmChannel_7/PwmChannelId - 7 
      | PwmChannel_7/PwmDutycycleDefault - 0 
      | PwmChannel_7/PwmHwChannel - /Pwm/Pwm/PwmChannelConfigSet/PwmEmios_1/PwmEmiosChannels_22 
      | PwmChannel_7/PwmIdleState - PWM_LOW 
      | PwmChannel_7/PwmMcuClockReferencePoint - /Mcu/Mcu/McuModuleConfiguration/McuClockSettingConfig_0/CORE_CLK 
      | PwmChannel_7/PwmNotification - PwmChannel_7_Callback 
      | PwmChannel_7/PwmPeriodDefault - 16000.0 
      | PwmChannel_7/PwmPeriodInTicks - true 
      | PwmChannel_7/PwmPolarity - PWM_HIGH 
      | PwmChannel_8/Index - 8 
      | PwmChannel_8/PwmChannelId - 8 
      | PwmChannel_8/PwmDutycycleDefault - 0 
      | PwmChannel_8/PwmHwChannel - /Pwm/Pwm/PwmChannelConfigSet/PwmEmios_2/PwmEmiosChannels_7 
      | PwmChannel_8/PwmIdleState - PWM_LOW 
      | PwmChannel_8/PwmMcuClockReferencePoint - /Mcu/Mcu/McuModuleConfiguration/McuClockSettingConfig_0/CORE_CLK 
      | PwmChannel_8/PwmNotification - PwmChannel_8_Callback 
      | PwmChannel_8/PwmPeriodDefault - 40000 
      | PwmChannel_8/PwmPeriodInTicks - true 
      | PwmChannel_8/PwmPolarity - PWM_HIGH 
      | PwmConfigurationOfOptApiServices - PwmConfigurationOfOptApiServices 
      | PwmConfigurationOfOptApiServices/PwmDeInitApi - true 
      | PwmConfigurationOfOptApiServices/PwmEmiosFastUpdateApi - true 
      | PwmConfigurationOfOptApiServices/PwmEnableMaskOutputs - false 
      | PwmConfigurationOfOptApiServices/PwmGetChannelStateApi - true 
      | PwmConfigurationOfOptApiServices/PwmGetOutputState - true 
      | PwmConfigurationOfOptApiServices/PwmSetChannelDeadTime - true 
      | PwmConfigurationOfOptApiServices/PwmSetChannelOutputApi - true 
      | PwmConfigurationOfOptApiServices/PwmSetCounterBusApi - true 
      | PwmConfigurationOfOptApiServices/PwmSetDutyCycle - true 
      | PwmConfigurationOfOptApiServices/PwmSetDutyCycle_NoUpdate - false 
      | PwmConfigurationOfOptApiServices/PwmSetDutyPhaseShift - false 
      | PwmConfigurationOfOptApiServices/PwmSetOutputToIdle - true 
      | PwmConfigurationOfOptApiServices/PwmSetPeriodAndDuty - true 
      | PwmConfigurationOfOptApiServices/PwmSetPeriodAndDuty_NoUpdate - false 
      | PwmConfigurationOfOptApiServices/PwmSetTriggerDelayApi - true 
      | PwmConfigurationOfOptApiServices/PwmVersionInfoApi - true 
      | PwmEmios - PwmEmios_0 PwmEmios_1 PwmEmios_2 
      | PwmEmios_0/Index - 0 
      | PwmEmios_0/PwmEmiosChannels - PwmEmiosChannels_17 PwmEmiosChannels_9 
      | PwmEmios_0/PwmEmiosChannels_17/EmiosChCounterBus - EMIOS_PWM_IP_BUS_A 
      | PwmEmios_0/PwmEmiosChannels_17/EmiosChDeadtime - 0 
      | PwmEmios_0/PwmEmiosChannels_17/EmiosChFlagGeneration - Trailing_Edge 
      | PwmEmios_0/PwmEmiosChannels_17/EmiosChFreeze - false 
      | PwmEmios_0/PwmEmiosChannels_17/EmiosChId - CH_17 
      | PwmEmios_0/PwmEmiosChannels_17/EmiosChInterrupt - EMIOS_PWM_IP_INTERRUPT_REQUEST 
      | PwmEmios_0/PwmEmiosChannels_17/EmiosChMode - EMIOS_PWM_IP_MODE_OPWMB 
      | PwmEmios_0/PwmEmiosChannels_17/EmiosChOutputDisable - EMIOS_PWM_IP_OUTPUT_DISABLE_NONE 
      | PwmEmios_0/PwmEmiosChannels_17/EmiosChPhaseShift - 0 
      | PwmEmios_0/PwmEmiosChannels_17/EmiosChPrescaler - EMIOS_PWM_IP_CLOCK_DIV_2 
      | PwmEmios_0/PwmEmiosChannels_17/EmiosChPrescalerAlternate - EMIOS_PWM_IP_CLOCK_DIV_1 
      | PwmEmios_0/PwmEmiosChannels_17/EmiosChPrescalerSource - EMIOS_PWM_IP_PS_SRC_MODULE_CLOCK 
      | PwmEmios_0/PwmEmiosChannels_17/EmiosChTrigger - 0 
      | PwmEmios_0/PwmEmiosChannels_17/Index - 1 
      | PwmEmios_0/PwmEmiosChannels_17/PwmEmiosBusRef - /Mcl/Mcl/MclConfig/EmiosCommon_0/EmiosMclMasterBus_0 
      | PwmEmios_0/PwmEmiosChannels_9/EmiosChCounterBus - EMIOS_PWM_IP_BUS_A 
      | PwmEmios_0/PwmEmiosChannels_9/EmiosChDeadtime - 0 
      | PwmEmios_0/PwmEmiosChannels_9/EmiosChFlagGeneration - Trailing_Edge 
      | PwmEmios_0/PwmEmiosChannels_9/EmiosChFreeze - false 
      | PwmEmios_0/PwmEmiosChannels_9/EmiosChId - CH_9 
      | PwmEmios_0/PwmEmiosChannels_9/EmiosChInterrupt - EMIOS_PWM_IP_INTERRUPT_REQUEST 
      | PwmEmios_0/PwmEmiosChannels_9/EmiosChMode - EMIOS_PWM_IP_MODE_OPWMB 
      | PwmEmios_0/PwmEmiosChannels_9/EmiosChOutputDisable - EMIOS_PWM_IP_OUTPUT_DISABLE_NONE 
      | PwmEmios_0/PwmEmiosChannels_9/EmiosChPhaseShift - 0 
      | PwmEmios_0/PwmEmiosChannels_9/EmiosChPrescaler - EMIOS_PWM_IP_CLOCK_DIV_1 
      | PwmEmios_0/PwmEmiosChannels_9/EmiosChPrescalerAlternate - EMIOS_PWM_IP_CLOCK_DIV_1 
      | PwmEmios_0/PwmEmiosChannels_9/EmiosChPrescalerSource - EMIOS_PWM_IP_PS_SRC_MODULE_CLOCK 
      | PwmEmios_0/PwmEmiosChannels_9/EmiosChTrigger - 0 
      | PwmEmios_0/PwmEmiosChannels_9/Index - 0 
      | PwmEmios_0/PwmEmiosChannels_9/PwmEmiosBusRef - /Mcl/Mcl/MclConfig/EmiosCommon_0/EmiosMclMasterBus_0 
      | PwmEmios_0/PwmHwInstance - Emios_0 
      | PwmEmios_1/Index - 1 
      | PwmEmios_1/PwmEmiosChannels - PwmEmiosChannels_0 PwmEmiosChannels_1 PwmEmiosChannels_19 PwmEmiosChannels_20 PwmEmiosChannels_21 PwmEmiosChannels_22 
      | PwmEmios_1/PwmEmiosChannels_0/EmiosChCounterBus - EMIOS_PWM_IP_BUS_A 
      | PwmEmios_1/PwmEmiosChannels_0/EmiosChDeadtime - 0 
      | PwmEmios_1/PwmEmiosChannels_0/EmiosChFlagGeneration - Trailing_Edge 
      | PwmEmios_1/PwmEmiosChannels_0/EmiosChFreeze - false 
      | PwmEmios_1/PwmEmiosChannels_0/EmiosChId - CH_0 
      | PwmEmios_1/PwmEmiosChannels_0/EmiosChInterrupt - EMIOS_PWM_IP_INTERRUPT_REQUEST 
      | PwmEmios_1/PwmEmiosChannels_0/EmiosChMode - EMIOS_PWM_IP_MODE_OPWMB 
      | PwmEmios_1/PwmEmiosChannels_0/EmiosChOutputDisable - EMIOS_PWM_IP_OUTPUT_DISABLE_NONE 
      | PwmEmios_1/PwmEmiosChannels_0/EmiosChPhaseShift - 0 
      | PwmEmios_1/PwmEmiosChannels_0/EmiosChPrescaler - EMIOS_PWM_IP_CLOCK_DIV_1 
      | PwmEmios_1/PwmEmiosChannels_0/EmiosChPrescalerAlternate - EMIOS_PWM_IP_CLOCK_DIV_1 
      | PwmEmios_1/PwmEmiosChannels_0/EmiosChPrescalerSource - EMIOS_PWM_IP_PS_SRC_MODULE_CLOCK 
      | PwmEmios_1/PwmEmiosChannels_0/EmiosChTrigger - 0 
      | PwmEmios_1/PwmEmiosChannels_0/Index - 2 
      | PwmEmios_1/PwmEmiosChannels_0/PwmEmiosBusRef - /Mcl/Mcl/MclConfig/EmiosCommon_1/EmiosMclMasterBus_0 
      | PwmEmios_1/PwmEmiosChannels_1/EmiosChCounterBus - EMIOS_PWM_IP_BUS_A 
      | PwmEmios_1/PwmEmiosChannels_1/EmiosChDeadtime - 0 
      | PwmEmios_1/PwmEmiosChannels_1/EmiosChFlagGeneration - Trailing_Edge 
      | PwmEmios_1/PwmEmiosChannels_1/EmiosChFreeze - false 
      | PwmEmios_1/PwmEmiosChannels_1/EmiosChId - CH_1 
      | PwmEmios_1/PwmEmiosChannels_1/EmiosChInterrupt - EMIOS_PWM_IP_INTERRUPT_REQUEST 
      | PwmEmios_1/PwmEmiosChannels_1/EmiosChMode - EMIOS_PWM_IP_MODE_OPWMB 
      | PwmEmios_1/PwmEmiosChannels_1/EmiosChOutputDisable - EMIOS_PWM_IP_OUTPUT_DISABLE_NONE 
      | PwmEmios_1/PwmEmiosChannels_1/EmiosChPhaseShift - 0 
      | PwmEmios_1/PwmEmiosChannels_1/EmiosChPrescaler - EMIOS_PWM_IP_CLOCK_DIV_1 
      | PwmEmios_1/PwmEmiosChannels_1/EmiosChPrescalerAlternate - EMIOS_PWM_IP_CLOCK_DIV_1 
      | PwmEmios_1/PwmEmiosChannels_1/EmiosChPrescalerSource - EMIOS_PWM_IP_PS_SRC_MODULE_CLOCK 
      | PwmEmios_1/PwmEmiosChannels_1/EmiosChTrigger - 0 
      | PwmEmios_1/PwmEmiosChannels_1/Index - 3 
      | PwmEmios_1/PwmEmiosChannels_1/PwmEmiosBusRef - /Mcl/Mcl/MclConfig/EmiosCommon_1/EmiosMclMasterBus_0 
      | PwmEmios_1/PwmEmiosChannels_19/EmiosChCounterBus - EMIOS_PWM_IP_BUS_A 
      | PwmEmios_1/PwmEmiosChannels_19/EmiosChDeadtime - 0 
      | PwmEmios_1/PwmEmiosChannels_19/EmiosChFlagGeneration - Trailing_Edge 
      | PwmEmios_1/PwmEmiosChannels_19/EmiosChFreeze - false 
      | PwmEmios_1/PwmEmiosChannels_19/EmiosChId - CH_19 
      | PwmEmios_1/PwmEmiosChannels_19/EmiosChInterrupt - EMIOS_PWM_IP_INTERRUPT_REQUEST 
      | PwmEmios_1/PwmEmiosChannels_19/EmiosChMode - EMIOS_PWM_IP_MODE_OPWMB 
      | PwmEmios_1/PwmEmiosChannels_19/EmiosChOutputDisable - EMIOS_PWM_IP_OUTPUT_DISABLE_NONE 
      | PwmEmios_1/PwmEmiosChannels_19/EmiosChPhaseShift - 0 
      | PwmEmios_1/PwmEmiosChannels_19/EmiosChPrescaler - EMIOS_PWM_IP_CLOCK_DIV_1 
      | PwmEmios_1/PwmEmiosChannels_19/EmiosChPrescalerAlternate - EMIOS_PWM_IP_CLOCK_DIV_1 
      | PwmEmios_1/PwmEmiosChannels_19/EmiosChPrescalerSource - EMIOS_PWM_IP_PS_SRC_MODULE_CLOCK 
      | PwmEmios_1/PwmEmiosChannels_19/EmiosChTrigger - 0 
      | PwmEmios_1/PwmEmiosChannels_19/Index - 0 
      | PwmEmios_1/PwmEmiosChannels_19/PwmEmiosBusRef - /Mcl/Mcl/MclConfig/EmiosCommon_1/EmiosMclMasterBus_0 
      | PwmEmios_1/PwmEmiosChannels_20/EmiosChCounterBus - EMIOS_PWM_IP_BUS_A 
      | PwmEmios_1/PwmEmiosChannels_20/EmiosChDeadtime - 0 
      | PwmEmios_1/PwmEmiosChannels_20/EmiosChFlagGeneration - Trailing_Edge 
      | PwmEmios_1/PwmEmiosChannels_20/EmiosChFreeze - false 
      | PwmEmios_1/PwmEmiosChannels_20/EmiosChId - CH_20 
      | PwmEmios_1/PwmEmiosChannels_20/EmiosChInterrupt - EMIOS_PWM_IP_INTERRUPT_REQUEST 
      | PwmEmios_1/PwmEmiosChannels_20/EmiosChMode - EMIOS_PWM_IP_MODE_OPWMB 
      | PwmEmios_1/PwmEmiosChannels_20/EmiosChOutputDisable - EMIOS_PWM_IP_OUTPUT_DISABLE_NONE 
      | PwmEmios_1/PwmEmiosChannels_20/EmiosChPhaseShift - 0 
      | PwmEmios_1/PwmEmiosChannels_20/EmiosChPrescaler - EMIOS_PWM_IP_CLOCK_DIV_1 
      | PwmEmios_1/PwmEmiosChannels_20/EmiosChPrescalerAlternate - EMIOS_PWM_IP_CLOCK_DIV_1 
      | PwmEmios_1/PwmEmiosChannels_20/EmiosChPrescalerSource - EMIOS_PWM_IP_PS_SRC_MODULE_CLOCK 
      | PwmEmios_1/PwmEmiosChannels_20/EmiosChTrigger - 0 
      | PwmEmios_1/PwmEmiosChannels_20/Index - 1 
      | PwmEmios_1/PwmEmiosChannels_20/PwmEmiosBusRef - /Mcl/Mcl/MclConfig/EmiosCommon_1/EmiosMclMasterBus_0 
      | PwmEmios_1/PwmEmiosChannels_21/EmiosChCounterBus - EMIOS_PWM_IP_BUS_A 
      | PwmEmios_1/PwmEmiosChannels_21/EmiosChDeadtime - 0 
      | PwmEmios_1/PwmEmiosChannels_21/EmiosChFlagGeneration - Trailing_Edge 
      | PwmEmios_1/PwmEmiosChannels_21/EmiosChFreeze - false 
      | PwmEmios_1/PwmEmiosChannels_21/EmiosChId - CH_21 
      | PwmEmios_1/PwmEmiosChannels_21/EmiosChInterrupt - EMIOS_PWM_IP_INTERRUPT_REQUEST 
      | PwmEmios_1/PwmEmiosChannels_21/EmiosChMode - EMIOS_PWM_IP_MODE_OPWMB 
      | PwmEmios_1/PwmEmiosChannels_21/EmiosChOutputDisable - EMIOS_PWM_IP_OUTPUT_DISABLE_NONE 
      | PwmEmios_1/PwmEmiosChannels_21/EmiosChPhaseShift - 0 
      | PwmEmios_1/PwmEmiosChannels_21/EmiosChPrescaler - EMIOS_PWM_IP_CLOCK_DIV_1 
      | PwmEmios_1/PwmEmiosChannels_21/EmiosChPrescalerAlternate - EMIOS_PWM_IP_CLOCK_DIV_1 
      | PwmEmios_1/PwmEmiosChannels_21/EmiosChPrescalerSource - EMIOS_PWM_IP_PS_SRC_MODULE_CLOCK 
      | PwmEmios_1/PwmEmiosChannels_21/EmiosChTrigger - 0 
      | PwmEmios_1/PwmEmiosChannels_21/Index - 4 
      | PwmEmios_1/PwmEmiosChannels_21/PwmEmiosBusRef - /Mcl/Mcl/MclConfig/EmiosCommon_1/EmiosMclMasterBus_0 
      | PwmEmios_1/PwmEmiosChannels_22/EmiosChCounterBus - EMIOS_PWM_IP_BUS_A 
      | PwmEmios_1/PwmEmiosChannels_22/EmiosChDeadtime - 0 
      | PwmEmios_1/PwmEmiosChannels_22/EmiosChFlagGeneration - Trailing_Edge 
      | PwmEmios_1/PwmEmiosChannels_22/EmiosChFreeze - false 
      | PwmEmios_1/PwmEmiosChannels_22/EmiosChId - CH_22 
      | PwmEmios_1/PwmEmiosChannels_22/EmiosChInterrupt - EMIOS_PWM_IP_INTERRUPT_REQUEST 
      | PwmEmios_1/PwmEmiosChannels_22/EmiosChMode - EMIOS_PWM_IP_MODE_OPWMB 
      | PwmEmios_1/PwmEmiosChannels_22/EmiosChOutputDisable - EMIOS_PWM_IP_OUTPUT_DISABLE_NONE 
      | PwmEmios_1/PwmEmiosChannels_22/EmiosChPhaseShift - 0 
      | PwmEmios_1/PwmEmiosChannels_22/EmiosChPrescaler - EMIOS_PWM_IP_CLOCK_DIV_1 
      | PwmEmios_1/PwmEmiosChannels_22/EmiosChPrescalerAlternate - EMIOS_PWM_IP_CLOCK_DIV_1 
      | PwmEmios_1/PwmEmiosChannels_22/EmiosChPrescalerSource - EMIOS_PWM_IP_PS_SRC_MODULE_CLOCK 
      | PwmEmios_1/PwmEmiosChannels_22/EmiosChTrigger - 0 
      | PwmEmios_1/PwmEmiosChannels_22/Index - 5 
      | PwmEmios_1/PwmEmiosChannels_22/PwmEmiosBusRef - /Mcl/Mcl/MclConfig/EmiosCommon_1/EmiosMclMasterBus_0 
      | PwmEmios_1/PwmHwInstance - Emios_1 
      | PwmEmios_2/Index - 2 
      | PwmEmios_2/PwmEmiosChannels - PwmEmiosChannels_7 
      | PwmEmios_2/PwmEmiosChannels_7/EmiosChCounterBus - EMIOS_PWM_IP_BUS_A 
      | PwmEmios_2/PwmEmiosChannels_7/EmiosChDeadtime - 0 
      | PwmEmios_2/PwmEmiosChannels_7/EmiosChFlagGeneration - Trailing_Edge 
      | PwmEmios_2/PwmEmiosChannels_7/EmiosChFreeze - false 
      | PwmEmios_2/PwmEmiosChannels_7/EmiosChId - CH_7 
      | PwmEmios_2/PwmEmiosChannels_7/EmiosChInterrupt - EMIOS_PWM_IP_INTERRUPT_REQUEST 
      | PwmEmios_2/PwmEmiosChannels_7/EmiosChMode - EMIOS_PWM_IP_MODE_OPWMB 
      | PwmEmios_2/PwmEmiosChannels_7/EmiosChOutputDisable - EMIOS_PWM_IP_OUTPUT_DISABLE_NONE 
      | PwmEmios_2/PwmEmiosChannels_7/EmiosChPhaseShift - 0 
      | PwmEmios_2/PwmEmiosChannels_7/EmiosChPrescaler - EMIOS_PWM_IP_CLOCK_DIV_2 
      | PwmEmios_2/PwmEmiosChannels_7/EmiosChPrescalerAlternate - EMIOS_PWM_IP_CLOCK_DIV_2 
      | PwmEmios_2/PwmEmiosChannels_7/EmiosChPrescalerSource - EMIOS_PWM_IP_PS_SRC_MODULE_CLOCK 
      | PwmEmios_2/PwmEmiosChannels_7/EmiosChTrigger - 0 
      | PwmEmios_2/PwmEmiosChannels_7/Index - 0 
      | PwmEmios_2/PwmEmiosChannels_7/PwmEmiosBusRef - /Mcl/Mcl/MclConfig/EmiosCommon_2/EmiosMclMasterBus_0 
      | PwmEmios_2/PwmHwInstance - Emios_2 
      | PwmEtpu - PwmChannelConfigSet 
      | PwmGeneral - PwmGeneral 
      | PwmGeneral/PwmDevErrorDetect - true 
      | PwmGeneral/PwmDutycycleUpdatedEndperiod - false 
      | PwmGeneral/PwmEnableDualClockMode - false 
      | PwmGeneral/PwmEnableUserModeSupport - false 
      | PwmGeneral/PwmIndex - 0 
      | PwmGeneral/PwmMultiChannelSync - false 
      | PwmGeneral/PwmMultipartitionEnabled - false 
      | PwmGeneral/PwmNotificationSupported - true 
      | PwmGeneral/PwmPeriodUpdatedEndperiod - true
      settings: SourceProductName=NXP Model-Based Design Toolbox for S32K3 MCUs
  Shift Arithmetic2 : ArithShift  BitShiftDirection=Right
  wires:
  Extract Bits22/1 -> Data Type Conversion23/1
  Data Type Conversion8/1 -> HSDl输出控制单元3/1(In1)
  Data Type Conversion23/1 -> HSDh输出控制单元5/2(In2)
  In5/1 -> Data Type Conversion28/1
  Data Type Conversion10/1 -> HSDl输出控制单元3/3(In3)
  Data Type Conversion3/1 -> HSDl输出控制单元1/4(In6)
  Data Type Conversion4/1 -> HSDl输出控制单元2/1(In1)
  Extract Bits8/1 -> Data Type Conversion10/1
  Extract Bits20/1 -> Data Type Conversion21/1
  Extract Bits2/1 -> Data Type Conversion4/1
  Data Type Conversion14/1 -> HSDl输出控制单元4/3(In3)
  Data Type Conversion6/1 -> HSDl输出控制单元2/3(In3)
  Extract Bits11/1 -> Data Type Conversion13/1
  Data Type Conversion15/1 -> HSDl输出控制单元4/4(In6)
  Extract Bits7/1 -> Data Type Conversion9/1
  Data Type Conversion27/1 -> HSDh输出控制单元3/2(In2)
  Extract Bits15/1 -> Data Type Conversion5/1
  Data Type Conversion22/1 -> HSDh输出控制单元5/1(In1)
  Data Type Conversion16/1 -> HSDl输出控制单元5/1(In1)
  Extract Bits5/1 -> Data Type Conversion7/1
  In2/1 -> Data Type Conversion25/1
  Data Type Conversion18/1 -> HSDl输出控制单元5/3(In3)
  Extract Bits26/1 -> Data Type Conversion18/1
  Extract Bits3/1 -> Data Type Conversion1/1
  In6/1 -> Data Type Conversion29/1
  Data Type Conversion/1 -> HSDl输出控制单元1/1(In1)
  Data Type Conversion24/1 -> HSDh输出控制单元3/1(In1)
  Data Type Conversion1/1 -> HSDl输出控制单元2/2(In2)
  Bitwise AND2/1 -> Shift Arithmetic2/1
  Extract Bits9/1 -> Data Type Conversion11/1
  Data Type Conversion9/1 -> HSDl输出控制单元3/2(In2)
  Extract Bits14/1 -> Data Type Conversion16/1
  Data Type Conversion21/1 -> HSDh输出控制单元2/1(In1)
  Data Type Conversion17/1 -> HSDl输出控制单元5/2(In2)
  Data Type Conversion19/1 -> HSDh输出控制单元1/1(In1)
  Data Type Conversion26/1 -> HSDh输出控制单元2/2(In2)
  Extract Bits21/1 -> Data Type Conversion22/1
  Shift Arithmetic2/1 -> Data Type Conversion/1
  Data Type Conversion5/1 -> HSDl输出控制单元5/4(In6)
  Extract Bits13/1 -> Data Type Conversion15/1
  Data Type Conversion7/1 -> HSDl输出控制单元2/4(In6)
  Extract Bits18/1 -> Data Type Conversion19/1
  Data Type Conversion11/1 -> HSDl输出控制单元3/4(In6)
  Extract Bits1/1 -> Data Type Conversion3/1
  Extract Bits4/1 -> Data Type Conversion6/1
  In1/1 -> Extract Bits26/1, Extract Bits15/1, Extract Bits18/1, Extract Bits22/1, Extract Bits21/1, Extract Bits23/1, Extract Bits20/1, Extract Bits19/1, Extract Bits17/1, Extract Bits14/1, Extract Bits13/1, Extract Bits12/1, Extract Bits11/1, Extract Bits10/1, Extract Bits9/1, Extract Bits8/1, Extract Bits7/1, Extract Bits6/1, Extract Bits5/1, Extract Bits4/1, Extract Bits3/1, Extract Bits2/1, Extract Bits/1, Bitwise AND2/1, Extract Bits1/1
  Extract Bits17/1 -> Data Type Conversion17/1
  Data Type Conversion2/1 -> HSDl输出控制单元1/3(In3)
  Data Type Conversion25/1 -> HSDl输出控制单元1/2(In2)
  Data Type Conversion29/1 -> HSDh输出控制单元4/2(In2)
  Extract Bits19/1 -> Data Type Conversion20/1
  Extract Bits/1 -> Data Type Conversion2/1
  Extract Bits6/1 -> Data Type Conversion8/1
  Data Type Conversion28/1 -> HSDh输出控制单元4/1(In1)
  Extract Bits12/1 -> Data Type Conversion14/1
  Data Type Conversion12/1 -> HSDl输出控制单元4/1(In1)
  In4/1 -> Data Type Conversion27/1
  Extract Bits23/1 -> Data Type Conversion24/1
  Extract Bits10/1 -> Data Type Conversion12/1
  In3/1 -> Data Type Conversion26/1
  Data Type Conversion13/1 -> HSDl输出控制单元4/2(In2)
  Data Type Conversion20/1 -> HSDh输出控制单元1/2(In2)

== system RBCM_Model/Subsystem13/Subsystem ==
  Action Port : ActionPort  ActionPortLabel=else
  HsdDriveCommand Struct1 : MATLAB Function  TreatAsAtomicUnit=on
  y : Outport
  wires:
  HsdDriveCommand Struct1/1(HsdDriveCommands) -> y/1

== system RBCM_Model/Subsystem13/Subsystem13 ==
  In1 : Inport
  Action Port : ActionPort  ActionPortLabel=if(u1 > 0)
  Out1 : Outport
  wires:
  In1/1 -> Out1/1

== system RBCM_Model/Subsystem5/Subsystem ==
  Action Port : ActionPort
  MATLAB Function : MATLAB Function  TreatAsAtomicUnit=on
  y : Outport
  wires:
  MATLAB Function/1(y) -> y/1

== system RBCM_Model/Subsystem5/Subsystem13 ==
  In1 : Inport
  Action Port : ActionPort
  Out1 : Outport
  wires:
  In1/1 -> Out1/1
